simulink model "hb_inverter"  (Simulink 6.1)
settings: Solver=ode23tb  StartTime=0.0  StopTime=0.1499  MaxStep=5e-5  RelTol=1e-3  AbsTol=.01
libraries: powerlib x7
settings Model: LastModifiedBy=ThinkPad
settings DebuggingCC: SolverPrmCheckMsg=warning

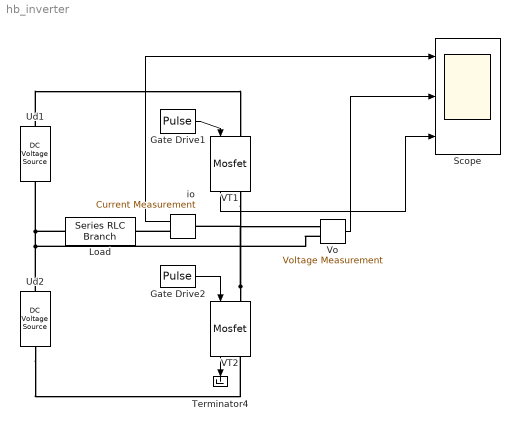
== system hb_inverter ==
  Gate Drive1 : DiscretePulseGenerator  PulseType=Time based  Period=0.02  PulseWidth=49.5
  Gate Drive2 : DiscretePulseGenerator  PulseType=Time based  Period=0.02  PulseWidth=49.5  PhaseDelay=0.01
  Load : powerlib/Elements/Series RLC Branch  Orientation=left  PhysicalDomain=powersysdomain  SubClassName=unknown  LeftPortType=p1  RightPortType=p1  LConnTagsString=__new0  RConnTagsString=__new0  Resistance=1  Inductance=0.01  Capacitance=inf  Measurements=None
  Scope : Scope  NumInputPorts=3
      settings: TimeRange=0.05  YMin=-100~-200~-50  YMax=100~200~250  SampleTime=2e-4
  Terminator4 : Terminator
      settings: Orientation=down
  Ud1 : powerlib/Electrical Sources/DC Voltage Source  Orientation=up  Amplitude=100  Measurements=None
  Ud2 : powerlib/Electrical Sources/DC Voltage Source  Orientation=up  Amplitude=100  Measurements=None
  VT1 : powerlib/Power Electronics/Mosfet  Orientation=down  Ron=0.01  Lon=1e-6  Rd=.01  IC=0  Rs=10  Cs=1e-6  Measurements=on
  VT2 : powerlib/Power Electronics/Mosfet  Orientation=down  Ron=0.01  Lon=1e-6  Rd=.01  IC=0  Rs=10  Cs=1e-6  Measurements=on
  Vo : powerlib/Measurements/Voltage Measurement  PhasorSimulation=off  OutputType=Complex  PSBequivalent=0
  io : powerlib/Measurements/Current Measurement  Orientation=left  PhasorSimulation=off  OutputType=Complex  PSBequivalent=0
  wires:
  Vo/1 -> Scope/2
  Gate Drive2/1 -> VT2/1
  Gate Drive1/1 -> VT1/1
  io/1 -> Scope/1
  VT1/1 -> Scope/3
  VT2/1 -> Terminator4/1
  connections:
  Ud2/LConn1 -- VT2/RConn1
  VT2/LConn1 -- io/LConn1 -- Vo/LConn1 -- VT1/RConn1
  Ud1/RConn1 -- VT1/LConn1
  Vo/LConn2 -- Load/RConn1 -- Ud1/LConn1 -- Ud2/RConn1
  io/RConn1 -- Load/LConn1
